simulink model "TestEulerWinkel"  (R2018a)
settings: Solver=VariableStepAuto  StartTime=0.0  StopTime=10.0  RelTol=1e-3
settings Model: Creator=martin  LastModifiedBy=martin

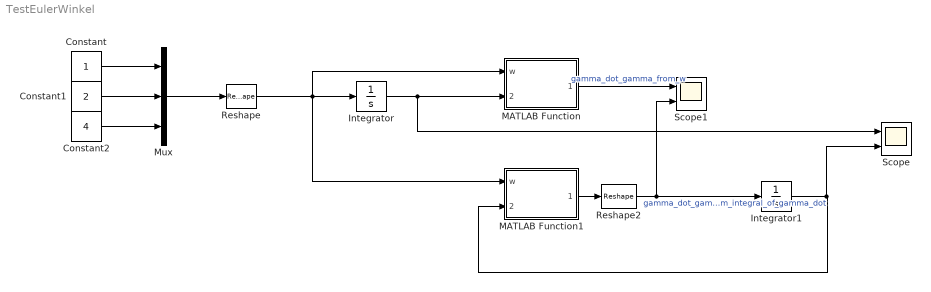
== system TestEulerWinkel ==
  Constant : Constant
  Constant1 : Constant  Value=2
  Constant2 : Constant  Value=4
  Integrator : Integrator
  Integrator1 : Integrator
  MATLAB Function : MATLAB Function  TreatAsAtomicUnit=on
  MATLAB Function1 : MATLAB Function  TreatAsAtomicUnit=on
  Mux : Mux  Inputs=3
  Reshape : Reshape  OutputDimensionality=Column vector (2-D)
  Reshape2 : Reshape  OutputDimensionality=Customize  OutputDimensions=[3,1]
  Scope : Scope  NumInputPorts=2
  Scope1 : Scope  NumInputPorts=2
  wires:
  Mux/1 -> Reshape/1
  Constant/1 -> Mux/1
  Constant1/1 -> Mux/2
  Constant2/1 -> Mux/3
  Reshape/1 -> MATLAB Function1/1(w), MATLAB Function/1(w), Integrator/1
  MATLAB Function1/1(gamma_dot) -> Reshape2/1
  Integrator1/1 -> MATLAB Function1/2(gamma), Scope/2
  Integrator/1 -> Scope/1, MATLAB Function/2(gamma)
  MATLAB Function/1(gamma_dot) -> Scope1/1  "gamma_dot_gamma_from_w"
  Reshape2/1 -> Scope1/2, Integrator1/1  "gamma_dot_gamma_from_integral_of_gamma_dot"

== matlab function TestEulerWinkel/MATLAB Function1 ==
  data: w input; gamma_dot output; gamma input
function gamma_dot = fcn(w,gamma)

phi = gamma(1);
theta = gamma(2);
psi = gamma(3);

gamma_dot = [0,	sin(phi)/(-sin(phi)^2*cos(theta)-cos(phi)^2*cos(theta)),	-cos(phi)/(-sin(phi)^2*cos(theta)-cos(phi)^2*cos(theta));
             0,	-(cos(phi)*cos(theta))/(-sin(phi)^2*cos(theta)-cos(phi)^2*cos(theta)),	-(sin(phi)*cos(theta))/(-sin(phi)^2*cos(theta)-cos(phi)^2*cos(theta));
             1,	-(sin(phi)*sin(theta))/(-sin(phi)^2*cos(theta)-cos(phi)^2*cos(theta)),	(cos(phi)*sin(theta))/(-sin(phi)^2*cos(theta)-cos(phi)^2*cos(theta))]*w;

== matlab function TestEulerWinkel/MATLAB Function ==
  data: w input; gamma_dot output; gamma input
function gamma_dot = fcn(w,gamma)

phi = gamma(1);
theta = gamma(2);
psi = gamma(3);

gamma_dot = [0,	sin(phi)/(-sin(phi)^2*cos(theta)-cos(phi)^2*cos(theta)),	-cos(phi)/(-sin(phi)^2*cos(theta)-cos(phi)^2*cos(theta));
             0,	-(cos(phi)*cos(theta))/(-sin(phi)^2*cos(theta)-cos(phi)^2*cos(theta)),	-(sin(phi)*cos(theta))/(-sin(phi)^2*cos(theta)-cos(phi)^2*cos(theta));
             1,	-(sin(phi)*sin(theta))/(-sin(phi)^2*cos(theta)-cos(phi)^2*cos(theta)),	(cos(phi)*sin(theta))/(-sin(phi)^2*cos(theta)-cos(phi)^2*cos(theta))]*w;
